simulink model "controlador_externo_y_observador"  (R2019a)
settings: Solver=VariableStepAuto  StartTime=0.0  StopTime=10.0  RelTol=1e-3
undefined symbols (not defined in the file): b_a, J_eq, k_sa, k_sia, ke_theta, ke_w
settings Model: Creator=miact  LastModifiedBy=pedro

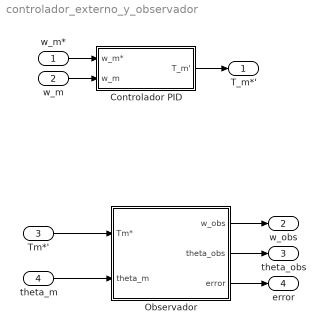
== system controlador_externo_y_observador ==
  w_m* : Inport
  w_m : Inport  Port=2
  Tm*' : Inport  Port=3
  theta_m : Inport  Port=4
  Controlador PID : Subsystem
  Observador : Subsystem
  T_m*' : Outport
  w_obs : Outport  Port=2
  theta_obs : Outport  Port=3
  error : Outport  Port=4
  wires:
  w_m*/1 -> Controlador PID/1(w_m*)
  w_m/1 -> Controlador PID/2(w_m)
  Controlador PID/1(T_m') -> T_m*'/1
  Tm*'/1 -> Observador/1(Tm*)
  theta_m/1 -> Observador/2(theta_m)
  Observador/1(w_obs) -> w_obs/1
  Observador/2(theta_obs) -> theta_obs/1
  Observador/3(error) -> error/1

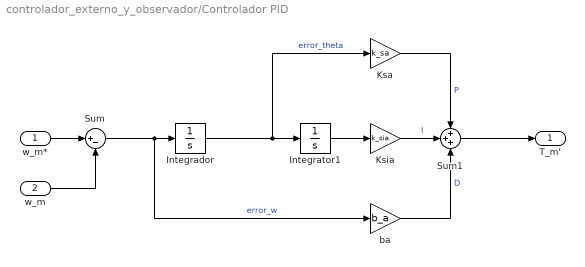
== system controlador_externo_y_observador/Controlador PID ==
  w_m* : Inport
  w_m : Inport  Port=2
  Integrador : Integrator
  Integrator1 : Integrator
  Ksa : Gain  Gain=k_sa
  Ksia : Gain  Gain=k_sia
  Sum : Sum  Inputs=|+-
  Sum1 : Sum  Inputs=+++
  ba : Gain  Gain=b_a
  T_m' : Outport
  wires:
  Sum/1 -> ba/1, Integrador/1  "error_w"
  w_m/1 -> Sum/2
  Sum1/1 -> T_m'/1
  Integrador/1 -> Integrator1/1, Ksa/1  "error_theta"
  ba/1 -> Sum1/3  "D"
  Integrator1/1 -> Ksia/1
  w_m*/1 -> Sum/1
  Ksia/1 -> Sum1/2  "I"
  Ksa/1 -> Sum1/1  "P"

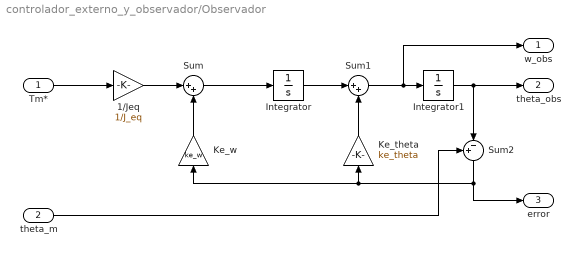
== system controlador_externo_y_observador/Observador ==
  Tm* : Inport
  theta_m : Inport  Port=2
  1/Jeq : Gain  Gain=1/J_eq
  Integrator : Integrator
  Integrator1 : Integrator
  Ke_theta : Gain  Gain=ke_theta
  Ke_w : Gain  Gain=ke_w
  Sum : Sum  Inputs=|++
  Sum1 : Sum  Inputs=|++
  Sum2 : Sum  Inputs=+-|
  w_obs : Outport
  theta_obs : Outport  Port=2
  error : Outport  Port=3
  wires:
  Integrator/1 -> Sum1/1
  Sum1/1 -> w_obs/1, Integrator1/1
  Sum2/1 -> error/1, Ke_w/1, Ke_theta/1
  Integrator1/1 -> Sum2/2, theta_obs/1
  Ke_w/1 -> Sum/2
  Tm*/1 -> 1/Jeq/1
  1/Jeq/1 -> Sum/1
  Sum/1 -> Integrator/1
  Ke_theta/1 -> Sum1/2
  theta_m/1 -> Sum2/1
